simulink model "123"  (R2013a)
settings: Solver=ode45  StartTime=0.0  StopTime=90  RelTol=1e-3
undefined symbols (not defined in the file): a, b, c, d
libraries: simulink x1
settings Model: Creator=user  LastModifiedBy=user

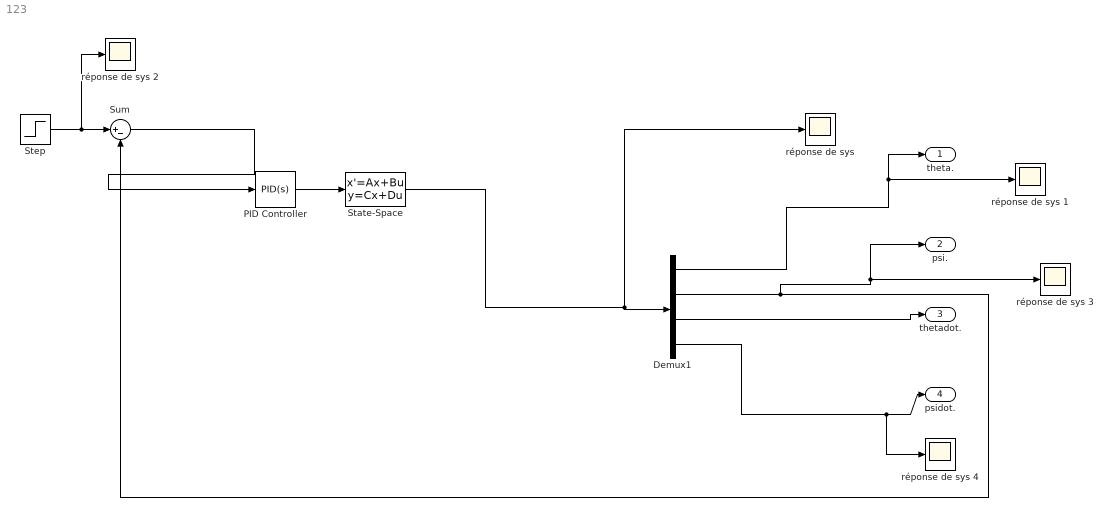
== system 123 ==
  Demux1 : Demux
  PID Controller : simulink/Continuous/PID Controller  Controller=PID  TimeDomain=Continuous-time  SampleTime=1  IntegratorMethod=Forward Euler  FilterMethod=Forward Euler  Form=Parallel  P=445.692952968504  I=2483.94170891961  D=19.2104645689599  N=297.531970793311  InitialConditionSource=internal  InitialConditionForIntegrator=0  InitialConditionForFilter=0  ExternalReset=none  LimitOutput=off  UpperSaturationLimit=inf  LowerSaturationLimit=-inf  LinearizeAsGain=on  AntiWindupMode=none  Kb=1  TrackingMode=off  Kt=1  PParamMin=[]  PParamMax=[]  IParamMin=[]  IParamMax=[]  DParamMin=[]  DParamMax=[]  NParamMin=[]  NParamMax=[]  KbParamMin=[]  KbParamMax=[]  KtParamMin=[]  KtParamMax=[]  POutMin=[]  POutMax=[]  IOutMin=[]  IOutMax=[]  DOutMin=[]  DOutMax=[]  NOutMin=[]  NOutMax=[]  KbOutMin=[]  KbOutMax=[]  KtOutMin=[]  KtOutMax=[]  IntegratorOutMin=[]  IntegratorOutMax=[]  FilterOutMin=[]  FilterOutMax=[]  SumOutMin=[]  SumOutMax=[]  SumI1OutMin=[]  SumI1OutMax=[]  SumI2OutMin=[]  SumI2OutMax=[]  SumI3OutMin=[]  SumI3OutMax=[]  SumDOutMin=[]  SumDOutMax=[]  SaturationOutMin=[]  SaturationOutMax=[]  IntegratorContinuousStateAttributes=''  IntegratorStateMustResolveToSignalObject=off  IntegratorRTWStateStorageClass=Auto  FilterContinuousStateAttributes=''  FilterStateMustResolveToSignalObject=off  FilterRTWStateStorageClass=Auto
  State-Space : StateSpace  A=a  B=b  C=c  D=d
  Step : Step  Time=4  After=20  SampleTime=0
  Sum : Sum  Inputs=|+-
  réponse de sys {,1..4} (5 alike) : Scope
      "réponse de sys " settings: YMin=-8.5e+07  YMax=5e+06
      réponse de sys 1 settings: YMin=-3.3e+07  YMax=-1.9e+07  SaveName=ScopeData3
      réponse de sys 3 settings: YMin=-5e+201  YMax=2e+201  SaveName=ScopeData2
      réponse de sys 4 settings: YMin=5.86516  YMax=5.8652  SaveName=ScopeData4
  theta. : Outport
  psi. : Outport  Port=2
  thetadot. : Outport  Port=3
  "psidot. " : Outport  Port=4
  wires:
  Demux1/2 -> Sum/2, réponse de sys 3/1, psi./1
  Demux1/3 -> thetadot./1
  Demux1/1 -> réponse de sys 1/1, theta./1
  State-Space/1 -> Demux1/1, "réponse de sys "/1
  Step/1 -> réponse de sys 2/1, Sum/1
  Sum/1 -> PID Controller/1
  Demux1/4 -> réponse de sys 4/1, "psidot. "/1
  PID Controller/1 -> State-Space/1
